simulink model "DDCU_wxt_v02_forA_LabviewV01"  (R2014a)
settings: Solver=FixedStepDiscrete  StartTime=0.0  StopTime=50  FixedStep=0.0005  RelTol=1e-3
InitFcn:
  | Veh_Par_wxt
values from neighbouring files (symbols this model uses):
  ag_thr = 0.4*g    (= 3.924)    [Veh_Par_wxt.m]
  B = 2.25    [Veh_Par_wxt.m]
  bra_pre_em = 12    [Veh_Par_wxt.m]
  bra_pre_gz2 = 12/3    (= 4)    [Veh_Par_wxt.m]
  bra_pre_gz34 = 12/3    (= 4)    [Veh_Par_wxt.m]
  bra_pre_yd = 12/2    (= 6)    [Veh_Par_wxt.m]
  brakepre_dem_data = [0 1 2 3 4 5 6 7 8 9 10 11 12]    [Veh_Par_wxt.m]
  brakeTrq_dem_data = [0 218.198 436.396 654.594 872.792 1090.99 1309.188 1527.386 1745.584 1963.782 2181.98 2400.178 2618.376]    [Veh_Par_wxt.m]
  bratrq_max = 4*2618.376    (= 10473.504)    [Veh_Par_wxt.m]
  eff_tran = 0.75    [Veh_Par_wxt.m]
  G = Mass*g    (= 36297)    [Veh_Par_wxt.m]
  kd1 = 1    [Veh_Par_wxt.m]
  kd2 = 1    [Veh_Par_wxt.m]
  kd3 = 1    [Veh_Par_wxt.m]
  ki1 = 1    [Veh_Par_wxt.m]
  ki2 = 1    [Veh_Par_wxt.m]
  ki3 = 1    [Veh_Par_wxt.m]
  kp1 = 1    [Veh_Par_wxt.m]
  kp2 = 1    [Veh_Par_wxt.m]
  kp3 = 1    [Veh_Par_wxt.m]
  L = 3.12    [Veh_Par_wxt.m]
  premax = 12    [Veh_Par_wxt.m]
  Radius = 0.20    (= 0.2)    [Veh_Par_wxt.m]
  s_opt_yi_add = 0.05    [Veh_Par_wxt.m]
  s_opt_zhuan_add = 0.05    [Veh_Par_wxt.m]
  spd_map_mot = [0 100 200 300 360 400 500 600 700 800 900]*tras_ratio    [Veh_Par_wxt.m]
  spdmax = 900*tras_ratio    (= 5580)    [Veh_Par_wxt.m]
  speed_thr_park = 5/3.6/Radius*30/pi    (= 66.3145596216)    [Veh_Par_wxt.m]
  tras_ratio = 6.2    [Veh_Par_wxt.m]
  trq_map_mot = [1200 1200 1200 1200 1200 1080 864 720 617 540 480]/tras_ratio    [Veh_Par_wxt.m]
  trqmax = 80    [Veh_Par_wxt.m]
  v_thr1_b = 5    [Veh_Par_wxt.m]
  v_thr2_b = 20    [Veh_Par_wxt.m]
  v_thr_park = 5    [Veh_Par_wxt.m]
undefined symbols (not defined in the file or in its folder): DiscIntNeverNeededParam
libraries: simulink x169, ec5744lib x9
(part 1 of 13)
settings Model: Creator=wxt  LastModifiedBy=wxt
settings OptimizationCC: InlineParams=on  InlineInvariantSignals=on  ExpressionFolding=off  RollThreshold=9  StateBitsets=on  DataBitsets=on  UseTempVars=on  ZeroExternalMemoryAtStartup=off  ZeroInternalMemoryAtStartup=off  EfficientFloat2IntCast=on  OptimizeModelRefInitCode=on  LifeSpan=1
settings DebuggingCC: InheritedTsInSrcMsg=none
settings HardwareCC: ProdLargestAtomicInteger=Long  ProdLargestAtomicFloat=Double  ProdIntDivRoundTo=Zero  ProdEndianess=BigEndian  ProdHWDeviceType=Freescale MPC5500
settings RTWCC: SystemTargetFile=ec5744.tlc  MakeCommand=make_rtw optimized_fixed_point=1  GenerateMakefile=off  TemplateMakefile=ec5744_lcc.tmf  PostCodeGenCommand=ec5744_pst_s2(buildInfo)  Description=Target for EC5744  GenerateReport=on  ProcessScript=ec5744_make_rtw_hook  IncludeHyperlinkInReport=on  LaunchReport=on
settings CodeAppCC: IgnoreCustomStorageClasses=off
settings STFCustomTargetCC: ModelReferenceCompliant=off  ConcurrentExecutionCompliant=off  IncludeMdlTerminateFcn=off  GeneratePreprocessorConditionals=Use local settings  CombineOutputUpdateFcns=on  SuppressErrorStatus=on  ERTCustomFileBanners=on  SupportContinuousTime=off  SupportNonInlinedSFcns=off  MATLABClassNameForMDSCustomization=Simulink.SoftwareTarget.ERTCustomization  GRTInterface=off  SystemTargetFile=ec5744.tlc
settings ERTTargetCC: GenerateSampleERTMain=off  ModelReferenceCompliant=off  IncludeMdlTerminateFcn=off  SuppressErrorStatus=on  GenerateASAP2=on  ERTSrcFileBannerTemplate=ec5744_code_template.cgt  ERTHdrFileBannerTemplate=ec5744_code_template.cgt  ERTDataSrcFileTemplate=ec5744_code_template.cgt  ERTDataHdrFileTemplate=ec5744_code_template.cgt  ERTCustomFileTemplate=ec5744_file_process.tlc

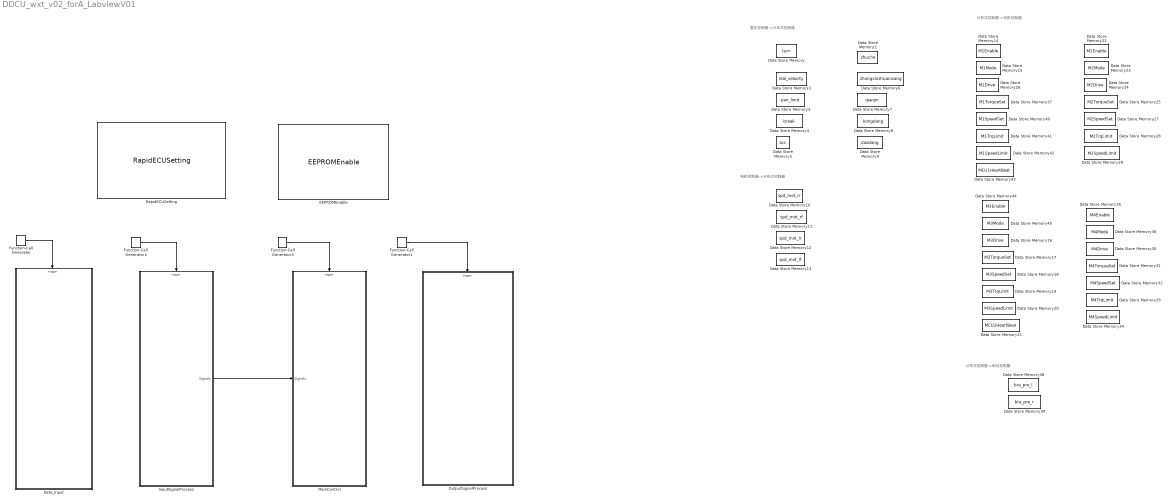
== system DDCU_wxt_v02_forA_LabviewV01 ==
  note: 电机控制器->分布式控制器
  note: 整车控制器->分布式控制器
  note: 分布式控制器->制动控制器
  note: 分布式控制器->电机控制器
  Data Store Memory : DataStoreMemory  DataStoreName=turn  ReadBeforeWriteMsg=warning  WriteAfterWriteMsg=warning  WriteAfterReadMsg=warning
  Data Store Memory1 : DataStoreMemory  DataStoreName=real_velocity  ReadBeforeWriteMsg=warning  WriteAfterWriteMsg=warning  WriteAfterReadMsg=warning
  Data Store Memory10 : DataStoreMemory  DataStoreName=spd_mot_rr  ReadBeforeWriteMsg=warning  WriteAfterWriteMsg=warning  WriteAfterReadMsg=warning
  Data Store Memory11 : DataStoreMemory  DataStoreName=spd_mot_rf  ReadBeforeWriteMsg=warning  WriteAfterWriteMsg=warning  WriteAfterReadMsg=warning
  Data Store Memory12 : DataStoreMemory  DataStoreName=spd_mot_lr  ReadBeforeWriteMsg=warning  WriteAfterWriteMsg=warning  WriteAfterReadMsg=warning
  Data Store Memory13 : DataStoreMemory  DataStoreName=spd_mot_lf  ReadBeforeWriteMsg=warning  WriteAfterWriteMsg=warning  WriteAfterReadMsg=warning
  Data Store Memory14 : DataStoreMemory  DataStoreName=M1Enable  ReadBeforeWriteMsg=warning  WriteAfterWriteMsg=warning  WriteAfterReadMsg=warning
  Data Store Memory15 : DataStoreMemory  DataStoreName=M1Mode  ReadBeforeWriteMsg=warning  WriteAfterWriteMsg=warning  WriteAfterReadMsg=warning
  Data Store Memory16 : DataStoreMemory  DataStoreName=M3Drive  ReadBeforeWriteMsg=warning  WriteAfterWriteMsg=warning  WriteAfterReadMsg=warning
  Data Store Memory17 : DataStoreMemory  DataStoreName=M3TorqueSet  ReadBeforeWriteMsg=warning  WriteAfterWriteMsg=warning  WriteAfterReadMsg=warning
  Data Store Memory18 : DataStoreMemory  DataStoreName=M3SpeedSet  ReadBeforeWriteMsg=warning  WriteAfterWriteMsg=warning  WriteAfterReadMsg=warning
  Data Store Memory19 : DataStoreMemory  DataStoreName=M3TrqLimit  ReadBeforeWriteMsg=warning  WriteAfterWriteMsg=warning  WriteAfterReadMsg=warning
  Data Store Memory2 : DataStoreMemory  DataStoreName=zhuche  ReadBeforeWriteMsg=warning  WriteAfterWriteMsg=warning  WriteAfterReadMsg=warning
  Data Store Memory20 : DataStoreMemory  DataStoreName=M3SpeedLimit  ReadBeforeWriteMsg=warning  WriteAfterWriteMsg=warning  WriteAfterReadMsg=warning
  Data Store Memory21 : DataStoreMemory  DataStoreName=MCU2HeartBeat  ReadBeforeWriteMsg=warning  WriteAfterWriteMsg=warning  WriteAfterReadMsg=warning
  Data Store Memory22 : DataStoreMemory  DataStoreName=M2Enable  ReadBeforeWriteMsg=warning  WriteAfterWriteMsg=warning  WriteAfterReadMsg=warning
  Data Store Memory23 : DataStoreMemory  DataStoreName=M2Mode  ReadBeforeWriteMsg=warning  WriteAfterWriteMsg=warning  WriteAfterReadMsg=warning
  Data Store Memory24 : DataStoreMemory  DataStoreName=M2Drive  ReadBeforeWriteMsg=warning  WriteAfterWriteMsg=warning  WriteAfterReadMsg=warning
  Data Store Memory25 : DataStoreMemory  DataStoreName=M2TorqueSet  ReadBeforeWriteMsg=warning  WriteAfterWriteMsg=warning  WriteAfterReadMsg=warning
  Data Store Memory26 : DataStoreMemory  DataStoreName=M1Drive  ReadBeforeWriteMsg=warning  WriteAfterWriteMsg=warning  WriteAfterReadMsg=warning
  Data Store Memory27 : DataStoreMemory  DataStoreName=M2SpeedSet  ReadBeforeWriteMsg=warning  WriteAfterWriteMsg=warning  WriteAfterReadMsg=warning
  Data Store Memory28 : DataStoreMemory  DataStoreName=M2TrqLimit  ReadBeforeWriteMsg=warning  WriteAfterWriteMsg=warning  WriteAfterReadMsg=warning
  Data Store Memory29 : DataStoreMemory  DataStoreName=M2SpeedLimit  ReadBeforeWriteMsg=warning  WriteAfterWriteMsg=warning  WriteAfterReadMsg=warning
  Data Store Memory3 : DataStoreMemory  DataStoreName=pwr_limit  ReadBeforeWriteMsg=warning  WriteAfterWriteMsg=warning  WriteAfterReadMsg=warning
  Data Store Memory30 : DataStoreMemory  DataStoreName=M4Drive  ReadBeforeWriteMsg=warning  WriteAfterWriteMsg=warning  WriteAfterReadMsg=warning
  Data Store Memory31 : DataStoreMemory  DataStoreName=M4TorqueSet  ReadBeforeWriteMsg=warning  WriteAfterWriteMsg=warning  WriteAfterReadMsg=warning
  Data Store Memory32 : DataStoreMemory  DataStoreName=M4SpeedSet  ReadBeforeWriteMsg=warning  WriteAfterWriteMsg=warning  WriteAfterReadMsg=warning
  Data Store Memory33 : DataStoreMemory  DataStoreName=M4TrqLimit  ReadBeforeWriteMsg=warning  WriteAfterWriteMsg=warning  WriteAfterReadMsg=warning
  Data Store Memory34 : DataStoreMemory  DataStoreName=M4SpeedLimit  ReadBeforeWriteMsg=warning  WriteAfterWriteMsg=warning  WriteAfterReadMsg=warning
  Data Store Memory35 : DataStoreMemory  DataStoreName=M4Enable  ReadBeforeWriteMsg=warning  WriteAfterWriteMsg=warning  WriteAfterReadMsg=warning
  Data Store Memory36 : DataStoreMemory  DataStoreName=M4Mode  ReadBeforeWriteMsg=warning  WriteAfterWriteMsg=warning  WriteAfterReadMsg=warning
  Data Store Memory37 : DataStoreMemory  DataStoreName=M1TorqueSet  ReadBeforeWriteMsg=warning  WriteAfterWriteMsg=warning  WriteAfterReadMsg=warning
  Data Store Memory38 : DataStoreMemory  DataStoreName=bra_pre_l  ReadBeforeWriteMsg=warning  WriteAfterWriteMsg=warning  WriteAfterReadMsg=warning
  Data Store Memory39 : DataStoreMemory  DataStoreName=bra_pre_r  ReadBeforeWriteMsg=warning  WriteAfterWriteMsg=warning  WriteAfterReadMsg=warning
  Data Store Memory4 : DataStoreMemory  DataStoreName=break  ReadBeforeWriteMsg=warning  WriteAfterWriteMsg=warning  WriteAfterReadMsg=warning
  Data Store Memory40 : DataStoreMemory  DataStoreName=M1SpeedSet  ReadBeforeWriteMsg=warning  WriteAfterWriteMsg=warning  WriteAfterReadMsg=warning
  Data Store Memory41 : DataStoreMemory  DataStoreName=M1TrqLimit  ReadBeforeWriteMsg=warning  WriteAfterWriteMsg=warning  WriteAfterReadMsg=warning
  Data Store Memory42 : DataStoreMemory  DataStoreName=M1SpeedLimit  ReadBeforeWriteMsg=warning  WriteAfterWriteMsg=warning  WriteAfterReadMsg=warning
  Data Store Memory43 : DataStoreMemory  DataStoreName=MCU1HeartBeat  ReadBeforeWriteMsg=warning  WriteAfterWriteMsg=warning  WriteAfterReadMsg=warning
  Data Store Memory44 : DataStoreMemory  DataStoreName=M3Enable  ReadBeforeWriteMsg=warning  WriteAfterWriteMsg=warning  WriteAfterReadMsg=warning
  Data Store Memory45 : DataStoreMemory  DataStoreName=M3Mode  ReadBeforeWriteMsg=warning  WriteAfterWriteMsg=warning  WriteAfterReadMsg=warning
  Data Store Memory5 : DataStoreMemory  DataStoreName=acc  ReadBeforeWriteMsg=warning  WriteAfterWriteMsg=warning  WriteAfterReadMsg=warning
  Data Store Memory6 : DataStoreMemory  DataStoreName=zhongxinzhuanxiang  ReadBeforeWriteMsg=warning  WriteAfterWriteMsg=warning  WriteAfterReadMsg=warning
  Data Store Memory7 : DataStoreMemory  DataStoreName=qianjin  ReadBeforeWriteMsg=warning  WriteAfterWriteMsg=warning  WriteAfterReadMsg=warning
  Data Store Memory8 : DataStoreMemory  DataStoreName=kongdang  ReadBeforeWriteMsg=warning  WriteAfterWriteMsg=warning  WriteAfterReadMsg=warning
  Data Store Memory9 : DataStoreMemory  DataStoreName=daodang  ReadBeforeWriteMsg=warning  WriteAfterWriteMsg=warning  WriteAfterReadMsg=warning
  Data_Input : Subsystem  TreatAsAtomicUnit=on
  EEPROMEnable : ec5744lib/RapidECU_U3/09MemoryManagement/EEPROMEnable  eepromenable=on
  Function-Call Generator{,1..3} (4 alike) : simulink/Ports & Subsystems/Function-Call Generator  sample_time=0.05  numberOfIterations=1
  InputSignalProcess : Subsystem
  MainControl : Subsystem
  OutputSignalProcess : Subsystem  TreatAsAtomicUnit=on
  RapidECUSetting : ec5744lib/RapidECU_U3/RapidECUSetting
      link override CAN: apdf=4  bpdf=4  cpdf=4  acmt=Extended(29-bit ID)  bcmt=Extended(29-bit ID)
      link override LIN: abrt=19200
  wires:
  Function-Call Generator/1 -> Data_Input/Trigger
  Function-Call Generator1/1 -> OutputSignalProcess/Trigger
  Function-Call Generator2/1 -> InputSignalProcess/Trigger
  InputSignalProcess/1(Signals) -> MainControl/1(Signals)
  Function-Call Generator3/1 -> MainControl/Trigger

== system DDCU_wxt_v02_forA_LabviewV01/Data_Input ==
  note: 电机控制器->分布式控制器
  note: 整车控制器->分布式控制器
  function : TriggerPort  TriggerType=function-call
  CANReceive : ec5744lib/RapidECU_U3/04CANCommunication/CANReceive  canmodule=0  canbuffer=0  canmessageid=hex2dec('1502C23A')  canmessagetype=Extended(29-bit ID)  datalength=8  sampletime=-1
  CANReceive1 : ec5744lib/RapidECU_U3/04CANCommunication/CANReceive  canmodule=0  canbuffer=1  canmessageid=hex2dec('0902C23A')  canmessagetype=Extended(29-bit ID)  datalength=8  sampletime=-1
  CANReceive2 : ec5744lib/RapidECU_U3/04CANCommunication/CANReceive  canmodule=0  canbuffer=2  canmessageid=hex2dec('0C0101F0')  canmessagetype=Extended(29-bit ID)  datalength=8  sampletime=-1
  Data Store Write : DataStoreWrite  DataStoreName=turn  DataStoreElements=turn
  Data Store Write1 : DataStoreWrite  DataStoreName=real_velocity
  Data Store Write10 : DataStoreWrite  DataStoreName=spd_mot_rr
  Data Store Write11 : DataStoreWrite  DataStoreName=spd_mot_rf
  Data Store Write12 : DataStoreWrite  DataStoreName=spd_mot_lr
  Data Store Write13 : DataStoreWrite  DialogController=Simulink.DDGSource  DataStoreName=spd_mot_lf  DataStoreElements=spd_mot_lf
  Data Store Write2 : DataStoreWrite  DataStoreName=pwr_limit
  Data Store Write3 : DataStoreWrite  DataStoreName=break
  Data Store Write4 : DataStoreWrite  DataStoreName=acc
  Data Store Write5 : DataStoreWrite  DataStoreName=zhuche
  Data Store Write6 : DataStoreWrite  DataStoreName=zhongxinzhuanxiang
  Data Store Write7 : DataStoreWrite  DataStoreName=qianjin
  Data Store Write8 : DataStoreWrite  DataStoreName=kongdang
  Data Store Write9 : DataStoreWrite  DataStoreName=daodang
  HCU1_VCU : Subsystem  TreatAsAtomicUnit=on
  HCU1_VCU1 : Subsystem  TreatAsAtomicUnit=on
  HCU2_VCU : Subsystem  TreatAsAtomicUnit=on
  Terminator{,1..5} (6 alike) : Terminator
  wires:
  CANReceive/1 -> HCU1_VCU/Trigger
  CANReceive/2 -> HCU1_VCU/1(In1)
  CANReceive/4 -> HCU1_VCU/2(In2)
  CANReceive/3 -> Terminator/1
  CANReceive/5 -> Terminator1/1
  HCU1_VCU/3(pwr_limit) -> Data Store Write2/1
  HCU1_VCU/2(real_velocity) -> Data Store Write1/1
  HCU1_VCU/4(break) -> Data Store Write3/1
  HCU1_VCU/1(turn) -> Data Store Write/1
  HCU1_VCU/5(acc) -> Data Store Write4/1
  CANReceive1/1 -> HCU2_VCU/Trigger
  CANReceive1/2 -> HCU2_VCU/1(In1)
  CANReceive1/4 -> HCU2_VCU/2(In2)
  CANReceive1/3 -> Terminator2/1
  CANReceive1/5 -> Terminator3/1
  HCU2_VCU/3(qianjin) -> Data Store Write7/1
  HCU2_VCU/4(kongdang) -> Data Store Write8/1
  HCU2_VCU/2(zhongxinzhuanxiang) -> Data Store Write6/1
  HCU2_VCU/1(zhuche) -> Data Store Write5/1
  HCU2_VCU/5(daodang) -> Data Store Write9/1
  CANReceive2/1 -> HCU1_VCU1/Trigger
  CANReceive2/2 -> HCU1_VCU1/1(In1)
  CANReceive2/4 -> HCU1_VCU1/2(In2)
  CANReceive2/3 -> Terminator4/1
  CANReceive2/5 -> Terminator5/1
  HCU1_VCU1/1(spd_mot_rr) -> Data Store Write10/1
  HCU1_VCU1/2(spd_mot_rf) -> Data Store Write11/1
  HCU1_VCU1/3(spd_mot_lr) -> Data Store Write12/1
  HCU1_VCU1/4(spd_mot_lf) -> Data Store Write13/1

== system DDCU_wxt_v02_forA_LabviewV01/InputSignalProcess ==
  note: 注：所有的单位转换都发生在此模块
      | 速度 km/h
      | 角速度 rpm
      | 加速度信号0-100
      | 制动信号0-100
      | 向左为正
      | 同时包括信号的一些简单处理，如根究摇杆位置，判断所需档位等
  function : TriggerPort  TriggerType=function-call
  Battery : Subsystem
  BraSystem : Subsystem
  Bus Creator : BusCreator  Inputs=6
  Constant{,1..3,6..8,15,17} (9 alike) : Constant  Value=0
  Constant{4..5,10,12} (4 alike) : Constant  Value=1000
  Constant{11,13..14,16} (4 alike) : Constant  Value=-1000
  Constant9 : Constant  Value=-80
  Data Store Read : DataStoreRead  DialogController=Simulink.DDGSource  DataStoreName=turn  DataStoreElements=turn
  Data Store Read1 : DataStoreRead  DataStoreName=pwr_limit
  Data Store Read10 : DataStoreRead  DataStoreName=spd_mot_rr
  Data Store Read11 : DataStoreRead  DataStoreName=spd_mot_rf
  Data Store Read12 : DataStoreRead  DataStoreName=spd_mot_lr
  Data Store Read13 : DataStoreRead  DataStoreName=spd_mot_lf  DataStoreElements=spd_mot_lf
  Data Store Read2 : DataStoreRead  DataStoreName=break
  Data Store Read3 : DataStoreRead  DataStoreName=acc
  Data Store Read4 : DataStoreRead  DataStoreName=real_velocity
  Data Store Read5 : DataStoreRead  DataStoreName=zhuche
  Data Store Read6 : DataStoreRead  DataStoreName=zhongxinzhuanxiang
  Data Store Read7 : DataStoreRead  DataStoreName=qianjin
  Data Store Read8 : DataStoreRead  DataStoreName=kongdang
  Data Store Read9 : DataStoreRead  DataStoreName=daodang
  DriveMotor : Subsystem
  IMU : Subsystem
  Signal Conversion : SignalConversion
  Subsystem : Subsystem
  Suspension : Subsystem
  YaoKong : Subsystem
  Signals : Outport
  wires:
  DriveMotor/1(DriveMotor) -> Bus Creator/2
  BraSystem/1(BraPre) -> Bus Creator/3
  YaoKong/1(YaoKong_dem) -> Bus Creator/1
  IMU/1(IMU) -> Bus Creator/4
  Suspension/1(Center_of_Mass) -> Bus Creator/5
  Battery/1(Bat) -> Bus Creator/6
  Constant8/1 -> Suspension/1(location_center)
  Constant9/1 -> Battery/2(pwr_chg_bat)
  Data Store Read1/1 -> Battery/1(pwr_dis_bat)  "pwr_limit"
  Data Store Read6/1 -> Subsystem/2(zhongxinzhuanxiang)  "zhongxinzhuanxiang"
  Data Store Read7/1 -> Subsystem/3(qianjin)  "qianjin"
  Data Store Read8/1 -> Subsystem/4(kongdang)  "kongdang"
  Data Store Read9/1 -> Subsystem/5(daodang)  "daodang"
  Subsystem/1(mode_dem) -> YaoKong/1(mode_dem)  "mode_dem"
  Data Store Read3/1 -> YaoKong/2(acc_dem)  "acc"
  Data Store Read/1 -> YaoKong/3(steer_dem)  "turn"
  Data Store Read2/1 -> YaoKong/4(brake_dem)  "breakyg"
  Data Store Read4/1 -> IMU/1(v_act)  "real_velocity"
  Data Store Read10/1 -> DriveMotor/16(speed_act_rr)  "spd_mot_rr"
  Data Store Read11/1 -> DriveMotor/11(speed_act_rf)  "spd_mot_rf"
  Data Store Read12/1 -> DriveMotor/6(speed_act_lr)  "spd_mot_lr"
  Data Store Read13/1 -> DriveMotor/1(speed_act_lf)  "spd_mot_lf"
  Bus Creator/1 -> Signal Conversion/1
  Constant/1 -> YaoKong/5(brake_emerg)
  Constant1/1 -> YaoKong/6(HAC)
  Constant6/1 -> BraSystem/2(BraPre_act_r), BraSystem/1(BraPre_act_l)
  Constant7/1 -> IMU/3(dis_north), IMU/4(dis_sky), IMU/5(hangxiangangle), IMU/6(fuyangangle), IMU/7(henggunangle), IMU/8(acc_x), IMU/9(acc_y), IMU/10(acc_z), IMU/11(jiaosudu_x), IMU/12(jiaosudu_y), IMU/13(jiaosudu_z), IMU/2(dis_east)
  Data Store Read5/1 -> Subsystem/1(zhuche)  "zhuche"
  Signal Conversion/1 -> Signals/1
  Constant2/1 -> DriveMotor/5(guzhang_lf)
  Constant10/1 -> DriveMotor/3(trqlimU_dig_lf)
  Constant11/1 -> DriveMotor/4(trqlimL_dig_lf)
  Constant3/1 -> DriveMotor/10(guzhang_lr)
  Constant12/1 -> DriveMotor/8(trqlimU_dig_lr)
  Constant13/1 -> DriveMotor/9(trqlimL_dig_lr)
  Constant15/1 -> DriveMotor/15(guzhang_rf)
  Constant4/1 -> DriveMotor/13(trqlimU_dig_rf)
  Constant14/1 -> DriveMotor/14(trqlimL_dig_rf)
  Constant17/1 -> DriveMotor/20(guzhang_rr)
  Constant5/1 -> DriveMotor/18(trqlimU_dig_rr)
  Constant16/1 -> DriveMotor/19(trqlimL_dig_rr)

== system DDCU_wxt_v02_forA_LabviewV01/MainControl ==
  Signals : Inport
  function : TriggerPort  TriggerType=function-call
  Scope : Scope
      settings: TimeRange=20  YMin=4  SaveName=ScopeData53
  SendOutPrepare : Subsystem
  To Workspace : ToWorkspace  VariableName=simout5  SaveFormat=Timeseries  SampleTime=-1
  mode_control : Subsystem
  mode_switch : Subsystem
  wires:
  Signals/1 -> mode_control/2(Signals), mode_switch/1(Signals)
  mode_switch/1(mode_dem_out) -> mode_control/1(mode_dem_out), Scope/1, To Workspace/1
  mode_control/1(com_dem) -> SendOutPrepare/1(com_dem)

== system DDCU_wxt_v02_forA_LabviewV01/OutputSignalProcess ==
  function : TriggerPort  TriggerType=function-call
  CANTransmit : ec5744lib/RapidECU_U3/04CANCommunication/CANTransmit  canmodule=0  canbuffer=8  canmessageid=hex2dec('0C01F001')  canmessagetype=Extended(29-bit ID)  datalength=8  sampletime=-1
  CANTransmit1 : ec5744lib/RapidECU_U3/04CANCommunication/CANTransmit  canmodule=0  canbuffer=9  canmessageid=hex2dec('0C01F002')  canmessagetype=Extended(29-bit ID)  datalength=8  sampletime=-1
  CANTransmit2 : ec5744lib/RapidECU_U3/04CANCommunication/CANTransmit  canmodule=0  canbuffer=10  canmessageid=hex2dec('804623A')  canmessagetype=Extended(29-bit ID)  datalength=8  sampletime=-1
  CANTransmit3 : ec5744lib/RapidECU_U3/04CANCommunication/CANTransmit  canmodule=0  canbuffer=11  canmessageid=hex2dec('0CF6EAF0')  canmessagetype=Extended(29-bit ID)  datalength=8  sampletime=-1
  Data Store Read : DataStoreRead  DataStoreName=M1Enable
  Data Store Read1 : DataStoreRead  DataStoreName=M1Mode
  Data Store Read10 : DataStoreRead  DataStoreName=M3Drive
  Data Store Read11 : DataStoreRead  DataStoreName=M3TorqueSet
  Data Store Read12 : DataStoreRead  DataStoreName=M3SpeedSet
  Data Store Read13 : DataStoreRead  DialogController=Simulink.DDGSource  DataStoreName=M3TrqLimit
  Data Store Read14 : DataStoreRead  DataStoreName=M3SpeedLimit
  Data Store Read15 : DataStoreRead  DataStoreName=MCU2HeartBeat
  Data Store Read16 : DataStoreRead  DataStoreName=M2Enable
  Data Store Read17 : DataStoreRead  DataStoreName=M2Mode
  Data Store Read18 : DataStoreRead  DataStoreName=M2Drive
  Data Store Read19 : DataStoreRead  DataStoreName=M2TorqueSet
  Data Store Read2 : DataStoreRead  DataStoreName=M1Drive
  Data Store Read20 : DataStoreRead  DataStoreName=M2SpeedSet
  Data Store Read21 : DataStoreRead  DataStoreName=M2TrqLimit
  Data Store Read22 : DataStoreRead  DataStoreName=M2SpeedLimit
  Data Store Read23 : DataStoreRead  DataStoreName=M4Drive
  Data Store Read24 : DataStoreRead  DataStoreName=M4TorqueSet
  Data Store Read25 : DataStoreRead  DataStoreName=M4SpeedSet
  Data Store Read26 : DataStoreRead  DataStoreName=M4TrqLimit
  Data Store Read27 : DataStoreRead  DataStoreName=M4SpeedLimit
  Data Store Read28 : DataStoreRead  DataStoreName=M4Enable
  Data Store Read29 : DataStoreRead  DataStoreName=M4Mode
  Data Store Read3 : DataStoreRead  DataStoreName=M1TorqueSet
  Data Store Read30 : DataStoreRead  DataStoreName=bra_pre_l
  Data Store Read31 : DataStoreRead  DataStoreName=bra_pre_r
  Data Store Read4 : DataStoreRead  DataStoreName=M1SpeedSet
  Data Store Read5 : DataStoreRead  DataStoreName=M1TrqLimit
  Data Store Read6 : DataStoreRead  DataStoreName=M1SpeedLimit
  Data Store Read7 : DataStoreRead  DataStoreName=MCU1HeartBeat
  Data Store Read8 : DataStoreRead  DataStoreName=M3Enable
  Data Store Read9 : DataStoreRead  DataStoreName=M3Mode
  Ground : Ground
  Ground1 : Ground
  Ground2 : Ground
  Terminator{,1..11} (12 alike) : Terminator
  VCU_ESC : Subsystem
  VCU_MCU1 : Subsystem
  VCU_MCU1_replace : Subsystem  Commented=on
  VCU_MCU2 : Subsystem
  VCU_MCU2_replace : Subsystem  Commented=on
  VCU_Park : Subsystem
  wires:
  Ground/1 -> VCU_Park/1(ParkEnable_in)
  Ground1/1 -> VCU_ESC/1(VVMS_BrkSts_flg_in)
  Ground2/1 -> VCU_ESC/2(VVMS_ParkSts_flg_in)
  VCU_MCU1/1(output) -> CANTransmit/1
  CANTransmit/1 -> Terminator/1
  VCU_MCU2/1(output) -> CANTransmit1/1
  CANTransmit1/1 -> Terminator1/1
  VCU_Park/1(output) -> CANTransmit2/1
  CANTransmit2/1 -> Terminator2/1
  VCU_ESC/1(output) -> CANTransmit3/1
  CANTransmit3/1 -> Terminator3/1
  Data Store Read4/1 -> Terminator4/1
  Data Store Read5/1 -> Terminator5/1
  Data Store Read20/1 -> Terminator6/1
  Data Store Read21/1 -> Terminator7/1
  Data Store Read12/1 -> Terminator8/1
  Data Store Read13/1 -> Terminator9/1
  Data Store Read25/1 -> Terminator10/1
  Data Store Read26/1 -> Terminator11/1
  Data Store Read7/1 -> VCU_MCU1/11(MCU1HeartBeat_in)
  Data Store Read19/1 -> VCU_MCU1/9(M2TorqueSet_in)  "M2TorqueSet"
  Data Store Read22/1 -> VCU_MCU1/10(M2SpeedLimit_in)
  Data Store Read6/1 -> VCU_MCU1/5(M1SpeedLimit_in)
  Data Store Read3/1 -> VCU_MCU1/4(M1TorqueSet_in)  "M1TorqueSet"
  Data Store Read16/1 -> VCU_MCU1/6(M2Enable_in)
  Data Store Read17/1 -> VCU_MCU1/7(M2Mode_in)
  Data Store Read18/1 -> VCU_MCU1/8(M2Drive_in)
  Data Store Read/1 -> VCU_MCU1/1(M1Enable_in)
  Data Store Read2/1 -> VCU_MCU1/3(M1Drive_in)
  Data Store Read1/1 -> VCU_MCU1/2(M1Mode_in)
  Data Store Read14/1 -> VCU_MCU2/5(M3SpeedLimit_in)
  Data Store Read11/1 -> VCU_MCU2/4(M3TorqueSet_in)  "M3TorqueSet"
  Data Store Read15/1 -> VCU_MCU2/11(MCU2HeartBeat_in)
  Data Store Read27/1 -> VCU_MCU2/10(M4SpeedLimit_in)
  Data Store Read10/1 -> VCU_MCU2/3(M3Drive_in)
  Data Store Read8/1 -> VCU_MCU2/1(M3Enable_in)
  Data Store Read9/1 -> VCU_MCU2/2(M3Mode_in)
  Data Store Read28/1 -> VCU_MCU2/6(M4Enable_in)
  Data Store Read24/1 -> VCU_MCU2/9(M4TorqueSet_in)  "M4TorqueSet"
  Data Store Read23/1 -> VCU_MCU2/8(M4Drive_in)
  Data Store Read29/1 -> VCU_MCU2/7(M4Mode_in)
  Data Store Read31/1 -> VCU_ESC/4(VVMS_BrkPSetRi_MPa_in)  "bra_pre_r"
  Data Store Read30/1 -> VCU_ESC/3(VVMS_BrkPSetLe_MPa_in)  "bra_pre_l"

== system DDCU_wxt_v02_forA_LabviewV01/Data_Input/HCU1_VCU ==
  In1 : Inport
  In2 : Inport  Port=2
  function : TriggerPort  TriggerType=function-call
  HCU1_VCU : Subsystem
  turn : Outport
  real_velocity : Outport  Port=2
  pwr_limit : Outport  Port=3
  break : Outport  Port=4
  acc : Outport  Port=5
  wires:
  In1/1 -> HCU1_VCU/Enable
  In2/1 -> HCU1_VCU/1(input)
  HCU1_VCU/3(pwr_limit_Out) -> pwr_limit/1
  HCU1_VCU/4(break_Out) -> break/1
  HCU1_VCU/2(real_velocity_Out) -> real_velocity/1
  HCU1_VCU/5(acc_Out) -> acc/1
  HCU1_VCU/1(turn_Out) -> turn/1

== system DDCU_wxt_v02_forA_LabviewV01/Data_Input/HCU1_VCU1 ==
  In1 : Inport
  In2 : Inport  Port=2
  function : TriggerPort  TriggerType=function-call
  MUC1_VCU1 : Subsystem
  spd_mot_rr : Outport
  spd_mot_rf : Outport  Port=2
  spd_mot_lr : Outport  Port=3
  spd_mot_lf : Outport  Port=4
  wires:
  In2/1 -> MUC1_VCU1/1(input)
  In1/1 -> MUC1_VCU1/Enable
  MUC1_VCU1/2(spd_mot_rf_Out) -> spd_mot_rf/1
  MUC1_VCU1/1(spd_mot_rr_Out) -> spd_mot_rr/1
  MUC1_VCU1/3(spd_mot_lr_Out) -> spd_mot_lr/1
  MUC1_VCU1/4(spd_mot_lf_Out) -> spd_mot_lf/1

== system DDCU_wxt_v02_forA_LabviewV01/Data_Input/HCU2_VCU ==
  In1 : Inport
  In2 : Inport  Port=2
  function : TriggerPort  TriggerType=function-call
  HCU2_VCU : Subsystem
  zhuche : Outport
  zhongxinzhuanxiang : Outport  Port=2
  qianjin : Outport  Port=3
  kongdang : Outport  Port=4
  daodang : Outport  Port=5
  wires:
  In2/1 -> HCU2_VCU/1(input)
  In1/1 -> HCU2_VCU/Enable
  HCU2_VCU/2(zhongxinzhuanxiang_Out) -> zhongxinzhuanxiang/1
  HCU2_VCU/3(qianjin_Out) -> qianjin/1
  HCU2_VCU/1(zhuche_Out) -> zhuche/1
  HCU2_VCU/4(kongdang_Out) -> kongdang/1
  HCU2_VCU/5(daodang_Out) -> daodang/1

== system DDCU_wxt_v02_forA_LabviewV01/InputSignalProcess/Battery ==
  pwr_dis_bat : Inport
  pwr_chg_bat : Inport  Port=2
  Bus Creator : BusCreator  Inputs=2
  Bat : Outport
  wires:
  pwr_dis_bat/1 -> Bus Creator/1  "pwr_dis_bat"
  Bus Creator/1 -> Bat/1  "Bat"
  pwr_chg_bat/1 -> Bus Creator/2  "pwr_chg_bat"

== system DDCU_wxt_v02_forA_LabviewV01/InputSignalProcess/BraSystem ==
  BraPre_act_l : Inport
  BraPre_act_r : Inport  Port=2
  Bus Creator : BusCreator  Inputs=2
  BraPre : Outport
  wires:
  BraPre_act_l/1 -> Bus Creator/1  "BraPre_act"
  Bus Creator/1 -> BraPre/1  "BraPre"
  BraPre_act_r/1 -> Bus Creator/2  "BraPre_act_r"

== system DDCU_wxt_v02_forA_LabviewV01/InputSignalProcess/DriveMotor ==
  speed_act_lf : Inport
  trq_act_lf : Inport  Port=2
  trqlimU_dig_lf : Inport  Port=3
  trqlimL_dig_lf : Inport  Port=4
  guzhang_lf : Inport  Port=5
  speed_act_lr : Inport  Port=6
  trq_act_lr : Inport  Port=7
  trqlimU_dig_lr : Inport  Port=8
  trqlimL_dig_lr : Inport  Port=9
  guzhang_lr : Inport  Port=10
  speed_act_rf : Inport  Port=11
  trq_act_rf : Inport  Port=12
  trqlimU_dig_rf : Inport  Port=13
  trqlimL_dig_rf : Inport  Port=14
  guzhang_rf : Inport  Port=15
  speed_act_rr : Inport  Port=16
  trq_act_rr : Inport  Port=17
  trqlimU_dig_rr : Inport  Port=18
  trqlimL_dig_rr : Inport  Port=19
  guzhang_rr : Inport  Port=20
  Bus Creator : BusCreator  Inputs=20
  DriveMotor : Outport
  wires:
  Bus Creator/1 -> DriveMotor/1  "DriveMotor"
  trqlimL_dig_lr/1 -> Bus Creator/9  "trqlimL_dig_lr"
  trq_act_lf/1 -> Bus Creator/2  "trq_act_lf"
  trq_act_lr/1 -> Bus Creator/7  "trq_act_lr"
  trqlimL_dig_lf/1 -> Bus Creator/4  "trqlimL_dig_lf"
  trqlimU_dig_lf/1 -> Bus Creator/3  "trqlimU_dig_lf"
  trqlimU_dig_lr/1 -> Bus Creator/8  "trqlimU_dig_lr"
  speed_act_lf/1 -> Bus Creator/1  "speed_act_lf"
  speed_act_lr/1 -> Bus Creator/6  "speed_act_lr"
  guzhang_rf/1 -> Bus Creator/15  "guzhang_rf"
  guzhang_lf/1 -> Bus Creator/5  "guzhang_lf"
  guzhang_lr/1 -> Bus Creator/10  "guzhang_lr"
  speed_act_rf/1 -> Bus Creator/11  "speed_act_rf"
  guzhang_rr/1 -> Bus Creator/20  "guzhang_rr"
  trq_act_rf/1 -> Bus Creator/12  "trq_act_rf"
  speed_act_rr/1 -> Bus Creator/16  "speed_act_rr"
  trqlimL_dig_rf/1 -> Bus Creator/14  "trqlimL_dig_rf"
  trq_act_rr/1 -> Bus Creator/17  "trq_act_rr"
  trqlimL_dig_rr/1 -> Bus Creator/19  "trqlimL_dig_rr"
  trqlimU_dig_rf/1 -> Bus Creator/13  "trqlimU_dig_rf"
  trqlimU_dig_rr/1 -> Bus Creator/18  "trqlimU_dig_rr"

== system DDCU_wxt_v02_forA_LabviewV01/InputSignalProcess/IMU ==
  v_act : Inport
  dis_east : Inport  Port=2
  dis_north : Inport  Port=3
  dis_sky : Inport  Port=4
  hangxiangangle : Inport  Port=5
  fuyangangle : Inport  Port=6
  henggunangle : Inport  Port=7
  acc_x : Inport  Port=8
  acc_y : Inport  Port=9
  acc_z : Inport  Port=10
  jiaosudu_x : Inport  Port=11
  jiaosudu_y : Inport  Port=12
  jiaosudu_z : Inport  Port=13
  Bus Creator : BusCreator  Inputs=13
  IMU : Outport
  wires:
  Bus Creator/1 -> IMU/1  "IMU"
  dis_east/1 -> Bus Creator/2  "dis_east"
  hangxiangangle/1 -> Bus Creator/5  "hangxiangangle"
  dis_north/1 -> Bus Creator/3  "dis_north"
  dis_sky/1 -> Bus Creator/4  "dis_sky"
  fuyangangle/1 -> Bus Creator/6  "fuyangangle"
  acc_y/1 -> Bus Creator/9  "acc_y"
  henggunangle/1 -> Bus Creator/7  "henggunangle"
  acc_x/1 -> Bus Creator/8  "acc_x"
  acc_z/1 -> Bus Creator/10  "acc_z"
  jiaosudu_z/1 -> Bus Creator/13  "jiaosudu_z"
  jiaosudu_x/1 -> Bus Creator/11  "jiaosudu_x"
  jiaosudu_y/1 -> Bus Creator/12  "jiaosudu_y"
  v_act/1 -> Bus Creator/1  "v_act"

== system DDCU_wxt_v02_forA_LabviewV01/InputSignalProcess/Subsystem ==
  zhuche : Inport
  zhongxinzhuanxiang : Inport  Port=2
  qianjin : Inport  Port=3
  kongdang : Inport  Port=4
  daodang : Inport  Port=5
  MATLAB Function : MATLAB Function  TreatAsAtomicUnit=on
  mode_dem : Outport
  wires:
  MATLAB Function/1(mode_dem) -> mode_dem/1
  zhuche/1 -> MATLAB Function/1(zhuche)
  zhongxinzhuanxiang/1 -> MATLAB Function/2(zhongxinzhuanxiang)
  qianjin/1 -> MATLAB Function/3(qianjin)
  kongdang/1 -> MATLAB Function/4(kongdang)
  daodang/1 -> MATLAB Function/5(daodang)

== system DDCU_wxt_v02_forA_LabviewV01/InputSignalProcess/Suspension ==
  location_center : Inport
  Bus Creator : BusCreator  Inputs=1
  Center_of_Mass : Outport
  wires:
  Bus Creator/1 -> Center_of_Mass/1  "Center_of_Mass"
  location_center/1 -> Bus Creator/1  "location_center"

== system DDCU_wxt_v02_forA_LabviewV01/InputSignalProcess/YaoKong ==
  note: 上坡辅助系统(Hill-start Assist Control，HAC)
  mode_dem : Inport
  acc_dem : Inport  Port=2
  steer_dem : Inport  Port=3
  brake_dem : Inport  Port=4
  brake_emerg : Inport  Port=5
  HAC : Inport  Port=6
  Bus Creator : BusCreator  Inputs=6
  YaoKong_dem : Outport
  wires:
  steer_dem/1 -> Bus Creator/3  "steer_dem"
  acc_dem/1 -> Bus Creator/2  "acc_dem"
  brake_dem/1 -> Bus Creator/4  "brake_dem"
  mode_dem/1 -> Bus Creator/1  "mode_dem"
  Bus Creator/1 -> YaoKong_dem/1  "YaoKong"
  brake_emerg/1 -> Bus Creator/5  "brake_emerg"
  HAC/1 -> Bus Creator/6  "HAC"

== system DDCU_wxt_v02_forA_LabviewV01/MainControl/SendOutPrepare ==
  com_dem : Inport
  Data Store Write : DataStoreWrite  DataStoreName=M1Enable
  Data Store Write1 : DataStoreWrite  DataStoreName=M1Mode
  Data Store Write10 : DataStoreWrite  DataStoreName=M3Drive
  Data Store Write11 : DataStoreWrite  DataStoreName=M3TorqueSet
  Data Store Write12 : DataStoreWrite  DataStoreName=M3SpeedSet
  Data Store Write13 : DataStoreWrite  DialogController=Simulink.DDGSource  DataStoreName=M3TrqLimit
  Data Store Write14 : DataStoreWrite  DataStoreName=M3SpeedLimit
  Data Store Write15 : DataStoreWrite  DataStoreName=MCU2HeartBeat
  Data Store Write16 : DataStoreWrite  DataStoreName=M2Enable
  Data Store Write17 : DataStoreWrite  DataStoreName=M2Mode
  Data Store Write18 : DataStoreWrite  DataStoreName=M2Drive
  Data Store Write19 : DataStoreWrite  DataStoreName=M2TorqueSet
  Data Store Write2 : DataStoreWrite  DataStoreName=M1Drive
  Data Store Write20 : DataStoreWrite  DataStoreName=M2SpeedSet
  Data Store Write21 : DataStoreWrite  DataStoreName=M2TrqLimit
  Data Store Write22 : DataStoreWrite  DataStoreName=M2SpeedLimit
  Data Store Write23 : DataStoreWrite  DataStoreName=M4Drive
  Data Store Write24 : DataStoreWrite  DataStoreName=M4TorqueSet
  Data Store Write25 : DataStoreWrite  DataStoreName=M4SpeedSet
  Data Store Write26 : DataStoreWrite  DataStoreName=M4TrqLimit
  Data Store Write27 : DataStoreWrite  DataStoreName=M4SpeedLimit
  Data Store Write28 : DataStoreWrite  DataStoreName=M4Enable
  Data Store Write29 : DataStoreWrite  DataStoreName=M4Mode
  Data Store Write3 : DataStoreWrite  DataStoreName=M1TorqueSet
  Data Store Write30 : DataStoreWrite  DataStoreName=bra_pre_l
  Data Store Write31 : DataStoreWrite  DataStoreName=bra_pre_r
  Data Store Write4 : DataStoreWrite  DataStoreName=M1SpeedSet
  Data Store Write5 : DataStoreWrite  DataStoreName=M1TrqLimit
  Data Store Write6 : DataStoreWrite  DataStoreName=M1SpeedLimit
  Data Store Write7 : DataStoreWrite  DataStoreName=MCU1HeartBeat
  Data Store Write8 : DataStoreWrite  DataStoreName=M3Enable
  Data Store Write9 : DataStoreWrite  DataStoreName=M3Mode
  Demux : Demux  Outputs=6
  Demux1 : Demux  Outputs=8
  Demux2 : Demux  Outputs=8
  Demux3 : Demux  Outputs=7
  Demux4 : Demux  Outputs=7
  Scope{,1..3} (4 alike) : Scope
      Scope2 settings: SaveName=ScopeData2
      Scope3 settings: SaveName=ScopeData3
  wires:
  Demux/1 -> Demux1/1
  Demux/2 -> Demux2/1
  Demux/3 -> Demux3/1
  Demux/4 -> Demux4/1
  Demux1/3 -> Data Store Write2/1
  Demux1/4 -> Scope/1, Data Store Write3/1
  Demux1/2 -> Data Store Write1/1
  Demux1/5 -> Data Store Write4/1
  Demux1/6 -> Data Store Write5/1
  Demux1/1 -> Data Store Write/1
  Demux1/7 -> Data Store Write6/1
  Demux1/8 -> Data Store Write7/1
  Demux2/7 -> Data Store Write14/1
  Demux2/6 -> Data Store Write13/1
  Demux2/1 -> Data Store Write8/1
  Demux2/8 -> Data Store Write15/1
  Demux2/5 -> Data Store Write12/1
  Demux2/2 -> Data Store Write9/1
  Demux2/4 -> Scope1/1, Data Store Write11/1
  Demux2/3 -> Data Store Write10/1
  Demux3/1 -> Data Store Write16/1
  Demux3/6 -> Data Store Write21/1
  Demux3/7 -> Data Store Write22/1
  Demux3/5 -> Data Store Write20/1
  Demux3/4 -> Scope2/1, Data Store Write19/1
  Demux3/2 -> Data Store Write17/1
  Demux3/3 -> Data Store Write18/1
  Demux4/1 -> Data Store Write28/1
  Demux4/2 -> Data Store Write29/1
  Demux4/3 -> Data Store Write23/1
  Demux4/4 -> Scope3/1, Data Store Write24/1
  Demux4/5 -> Data Store Write25/1
  Demux4/6 -> Data Store Write26/1
  Demux4/7 -> Data Store Write27/1
  Demux/5 -> Data Store Write30/1
  Demux/6 -> Data Store Write31/1
  com_dem/1 -> Demux/1

== system DDCU_wxt_v02_forA_LabviewV01/MainControl/mode_control ==
  mode_dem_out : Inport
  Signals : Inport  Port=2
  Multiport Switch : MultiPortSwitch  DataPortOrder=Zero-based contiguous  Inputs=6
  Park : Subsystem  TreatAsAtomicUnit=on
  Switch Case : SwitchCase  CaseConditions={0,1,2,3,4,5}  ShowDefaultCase=off
  backward : Subsystem  TreatAsAtomicUnit=on
  center_steer : Subsystem  TreatAsAtomicUnit=on
  emergency_stop : Subsystem  TreatAsAtomicUnit=on
  forward : Subsystem  TreatAsAtomicUnit=on
  neutral : Subsystem  TreatAsAtomicUnit=on
  com_dem : Outport
  wires:
  mode_dem_out/1 -> Multiport Switch/1, Switch Case/1
  Signals/1 -> backward/1(Signals), emergency_stop/1(Signals), center_steer/1(Signals), neutral/1(Signals), forward/1(Signals), Park/1(Signals)
  Switch Case/1 -> Park/Action
  Switch Case/6 -> emergency_stop/Action
  Switch Case/5 -> center_steer/Action
  Switch Case/4 -> backward/Action
  Switch Case/3 -> neutral/Action
  Switch Case/2 -> forward/Action
  Park/1(park_dem) -> Multiport Switch/2
  forward/1(forward_dem) -> Multiport Switch/3
  backward/1(backward_dem) -> Multiport Switch/5
  neutral/1(neutral_dem) -> Multiport Switch/4
  center_steer/1(center_steer_dem) -> Multiport Switch/6
  emergency_stop/1(emergency_stop_dem) -> Multiport Switch/7
  Multiport Switch/1 -> com_dem/1

== system DDCU_wxt_v02_forA_LabviewV01/MainControl/mode_switch ==
  Signals : Inport
  Abs{,1..3} (4 alike) : Abs
  Bus Selector : BusSelector  OutputSignals=YaoKong.mode_dem,YaoKong.brake_emerg,DriveMotor.speed_act_lf,DriveMotor.speed_act_lr,DriveMotor.speed_act_rf,DriveMotor.speed_act_rr,IMU.v_act
  Constant1 : Constant  Value=v_thr_park
  Constant2 : Constant  Value=speed_thr_park
  Memory : Memory  InheritSampleTime=on
  mode_switch : MATLAB Function  TreatAsAtomicUnit=on
  mode_dem_out : Outport
  wires:
  Memory/1 -> mode_switch/10(mode_dem_out_pre)
  Signals/1 -> Bus Selector/1
  Bus Selector/3 -> Abs/1  "<speed_act_lf>"
  Bus Selector/2 -> mode_switch/2(brake_emerg)  "<brake_emerg>"
  Bus Selector/1 -> mode_switch/1(mode_dem)  "<mode_dem>"
  Bus Selector/5 -> Abs2/1  "<speed_act_rf>"
  Bus Selector/4 -> Abs1/1  "<speed_act_lr>"
  Bus Selector/6 -> Abs3/1  "<speed_act_rr>"
  Bus Selector/7 -> mode_switch/7(v_act)  "<v_act>"
  mode_switch/1(mode_dem_out) -> mode_dem_out/1, Memory/1
  Constant2/1 -> mode_switch/9(speed_thr_park)
  Constant1/1 -> mode_switch/8(v_thr_park)
  Abs/1 -> mode_switch/3(speed_act_lf)
  Abs1/1 -> mode_switch/4(speed_act_lr)
  Abs2/1 -> mode_switch/5(speed_act_rf)
  Abs3/1 -> mode_switch/6(speed_act_rr)

== system DDCU_wxt_v02_forA_LabviewV01/OutputSignalProcess/VCU_ESC ==
  VVMS_BrkSts_flg_in : Inport
  VVMS_ParkSts_flg_in : Inport  Port=2
  VVMS_BrkPSetLe_MPa_in : Inport  Port=3
  VVMS_BrkPSetRi_MPa_in : Inport  Port=4
  Conv{1..8} (8 alike) : DataTypeConversion
  VCU_ESC_DLC : Constant  Value=8  OutDataTypeStr=uint8
  VCU_ESC_DLC_Out : Terminator
  VCU_ESC_ID : Constant  Value=2364992240  OutDataTypeStr=single
  VCU_ESC_ID_Out : Terminator
  VCU_ESC_mux : Mux  Inputs=8
  VVMS_BrkPSetLe_MPa : Subsystem
  VVMS_BrkPSetRi_MPa : Subsystem
  VVMS_BrkSts_flg : Subsystem
  VVMS_ParkSts_flg : Subsystem
  or{1..8} (8 alike) : simulink/Logic and Bit Operations/Bitwise Operator  logicop=OR  UseBitMask=off  NumInputPorts=4  BitMask=bin2dec('11011001')  BitMaskRealWorld=Stored Integer
  output : Outport
  wires:
  VCU_ESC_mux/1 -> output/1
  VVMS_BrkSts_flg/1(output1) -> or1/1
  VVMS_BrkSts_flg/2(output2) -> or2/1
  VVMS_BrkSts_flg/3(output3) -> or3/1
  VVMS_BrkSts_flg/4(output4) -> or4/1
  VVMS_BrkSts_flg/5(output5) -> or5/1
  VVMS_BrkSts_flg/6(output6) -> or6/1
  VVMS_BrkSts_flg/7(output7) -> or7/1
  VVMS_BrkSts_flg/8(output8) -> or8/1
  VVMS_ParkSts_flg/1(output1) -> or1/2
  VVMS_ParkSts_flg/2(output2) -> or2/2
  VVMS_ParkSts_flg/3(output3) -> or3/2
  VVMS_ParkSts_flg/4(output4) -> or4/2
  VVMS_ParkSts_flg/5(output5) -> or5/2
  VVMS_ParkSts_flg/6(output6) -> or6/2
  VVMS_ParkSts_flg/7(output7) -> or7/2
  VVMS_ParkSts_flg/8(output8) -> or8/2
  VVMS_BrkPSetRi_MPa/1(output1) -> or1/3
  VVMS_BrkPSetRi_MPa/2(output2) -> or2/3
  VVMS_BrkPSetRi_MPa/3(output3) -> or3/3
  VVMS_BrkPSetRi_MPa/4(output4) -> or4/3
  VVMS_BrkPSetRi_MPa/5(output5) -> or5/3
  VVMS_BrkPSetRi_MPa/6(output6) -> or6/3
  VVMS_BrkPSetRi_MPa/7(output7) -> or7/3
  VVMS_BrkPSetRi_MPa/8(output8) -> or8/3
  VVMS_BrkPSetLe_MPa/1(output1) -> or1/4
  VVMS_BrkPSetLe_MPa/2(output2) -> or2/4
  VVMS_BrkPSetLe_MPa/3(output3) -> or3/4
  VVMS_BrkPSetLe_MPa/4(output4) -> or4/4
  VVMS_BrkPSetLe_MPa/5(output5) -> or5/4
  VVMS_BrkPSetLe_MPa/6(output6) -> or6/4
  VVMS_BrkPSetLe_MPa/7(output7) -> or7/4
  VVMS_BrkPSetLe_MPa/8(output8) -> or8/4
  or1/1 -> Conv1/1
  Conv1/1 -> VCU_ESC_mux/1
  or2/1 -> Conv2/1
  Conv2/1 -> VCU_ESC_mux/2
  or3/1 -> Conv3/1
  Conv3/1 -> VCU_ESC_mux/3
  or4/1 -> Conv4/1
  Conv4/1 -> VCU_ESC_mux/4
  or5/1 -> Conv5/1
  Conv5/1 -> VCU_ESC_mux/5
  or6/1 -> Conv6/1
  Conv6/1 -> VCU_ESC_mux/6
  or7/1 -> Conv7/1
  Conv7/1 -> VCU_ESC_mux/7
  or8/1 -> Conv8/1
  Conv8/1 -> VCU_ESC_mux/8
  VCU_ESC_ID/1 -> VCU_ESC_ID_Out/1
  VCU_ESC_DLC/1 -> VCU_ESC_DLC_Out/1
  VVMS_BrkSts_flg_in/1 -> VVMS_BrkSts_flg/1(VVMS_BrkSts_flg)
  VVMS_ParkSts_flg_in/1 -> VVMS_ParkSts_flg/1(VVMS_ParkSts_flg)
  VVMS_BrkPSetRi_MPa_in/1 -> VVMS_BrkPSetRi_MPa/1(VVMS_BrkPSetRi_MPa)
  VVMS_BrkPSetLe_MPa_in/1 -> VVMS_BrkPSetLe_MPa/1(VVMS_BrkPSetLe_MPa)

== system DDCU_wxt_v02_forA_LabviewV01/OutputSignalProcess/VCU_MCU1 ==
  M1Enable_in : Inport
  M1Mode_in : Inport  Port=2
  M1Drive_in : Inport  Port=3
  M1TorqueSet_in : Inport  Port=4
  M1SpeedLimit_in : Inport  Port=5
  M2Enable_in : Inport  Port=6
  M2Mode_in : Inport  Port=7
  M2Drive_in : Inport  Port=8
  M2TorqueSet_in : Inport  Port=9
  M2SpeedLimit_in : Inport  Port=10
  MCU1HeartBeat_in : Inport  Port=11
  Conv{1..8} (8 alike) : DataTypeConversion
  M1Drive : Subsystem
  M1Enable : Subsystem
  M1Mode : Subsystem
  M1SpeedLimit : Subsystem
  M1TorqueSet : Subsystem
  M2Drive : Subsystem
  M2Enable : Subsystem
  M2Mode : Subsystem
  M2SpeedLimit : Subsystem
  M2TorqueSet : Subsystem
  MCU1HeartBeat : Subsystem
  VCU_MCU1_DLC : Constant  Value=8  OutDataTypeStr=uint8
  VCU_MCU1_DLC_Out : Terminator
  VCU_MCU1_ID : Constant  Value=2348937217  OutDataTypeStr=single
  VCU_MCU1_ID_Out : Terminator
  VCU_MCU1_mux : Mux  Inputs=8
  or{1..8} (8 alike) : simulink/Logic and Bit Operations/Bitwise Operator  logicop=OR  UseBitMask=off  NumInputPorts=11  BitMask=bin2dec('11011001')  BitMaskRealWorld=Stored Integer
  output : Outport
  wires:
  VCU_MCU1_mux/1 -> output/1
  MCU1HeartBeat/1(output1) -> or1/1
  MCU1HeartBeat/2(output2) -> or2/1
  MCU1HeartBeat/3(output3) -> or3/1
  MCU1HeartBeat/4(output4) -> or4/1
  MCU1HeartBeat/5(output5) -> or5/1
  MCU1HeartBeat/6(output6) -> or6/1
  MCU1HeartBeat/7(output7) -> or7/1
  MCU1HeartBeat/8(output8) -> or8/1
  M2TorqueSet/1(output1) -> or1/2
  M2TorqueSet/2(output2) -> or2/2
  M2TorqueSet/3(output3) -> or3/2
  M2TorqueSet/4(output4) -> or4/2
  M2TorqueSet/5(output5) -> or5/2
  M2TorqueSet/6(output6) -> or6/2
  M2TorqueSet/7(output7) -> or7/2
  M2TorqueSet/8(output8) -> or8/2
  M2SpeedLimit/1(output1) -> or1/3
  M2SpeedLimit/2(output2) -> or2/3
  M2SpeedLimit/3(output3) -> or3/3
  M2SpeedLimit/4(output4) -> or4/3
  M2SpeedLimit/5(output5) -> or5/3
  M2SpeedLimit/6(output6) -> or6/3
  M2SpeedLimit/7(output7) -> or7/3
  M2SpeedLimit/8(output8) -> or8/3
  M2Mode/1(output1) -> or1/4
  M2Mode/2(output2) -> or2/4
  M2Mode/3(output3) -> or3/4
  M2Mode/4(output4) -> or4/4
  M2Mode/5(output5) -> or5/4
  M2Mode/6(output6) -> or6/4
  M2Mode/7(output7) -> or7/4
  M2Mode/8(output8) -> or8/4
  M2Enable/1(output1) -> or1/5
  M2Enable/2(output2) -> or2/5
  M2Enable/3(output3) -> or3/5
  M2Enable/4(output4) -> or4/5
  M2Enable/5(output5) -> or5/5
  M2Enable/6(output6) -> or6/5
  M2Enable/7(output7) -> or7/5
  M2Enable/8(output8) -> or8/5
  M2Drive/1(output1) -> or1/6
  M2Drive/2(output2) -> or2/6
  M2Drive/3(output3) -> or3/6
  M2Drive/4(output4) -> or4/6
  M2Drive/5(output5) -> or5/6
  M2Drive/6(output6) -> or6/6
  M2Drive/7(output7) -> or7/6
  M2Drive/8(output8) -> or8/6
  M1TorqueSet/1(output1) -> or1/7
  M1TorqueSet/2(output2) -> or2/7
  M1TorqueSet/3(output3) -> or3/7
  M1TorqueSet/4(output4) -> or4/7
  M1TorqueSet/5(output5) -> or5/7
  M1TorqueSet/6(output6) -> or6/7
  M1TorqueSet/7(output7) -> or7/7
  M1TorqueSet/8(output8) -> or8/7
  M1SpeedLimit/1(output1) -> or1/8
  M1SpeedLimit/2(output2) -> or2/8
  M1SpeedLimit/3(output3) -> or3/8
  M1SpeedLimit/4(output4) -> or4/8
  M1SpeedLimit/5(output5) -> or5/8
  M1SpeedLimit/6(output6) -> or6/8
  M1SpeedLimit/7(output7) -> or7/8
  M1SpeedLimit/8(output8) -> or8/8
  M1Mode/1(output1) -> or1/9
  M1Mode/2(output2) -> or2/9
  M1Mode/3(output3) -> or3/9
  M1Mode/4(output4) -> or4/9
  M1Mode/5(output5) -> or5/9
  M1Mode/6(output6) -> or6/9
  M1Mode/7(output7) -> or7/9
  M1Mode/8(output8) -> or8/9
  M1Enable/1(output1) -> or1/10
  M1Enable/2(output2) -> or2/10
  M1Enable/3(output3) -> or3/10
  M1Enable/4(output4) -> or4/10
  M1Enable/5(output5) -> or5/10
  M1Enable/6(output6) -> or6/10
  M1Enable/7(output7) -> or7/10
  M1Enable/8(output8) -> or8/10
  M1Drive/1(output1) -> or1/11
  M1Drive/2(output2) -> or2/11
  M1Drive/3(output3) -> or3/11
  M1Drive/4(output4) -> or4/11
  M1Drive/5(output5) -> or5/11
  M1Drive/6(output6) -> or6/11
  M1Drive/7(output7) -> or7/11
  M1Drive/8(output8) -> or8/11
  or1/1 -> Conv1/1
  Conv1/1 -> VCU_MCU1_mux/1
  or2/1 -> Conv2/1
  Conv2/1 -> VCU_MCU1_mux/2
  or3/1 -> Conv3/1
  Conv3/1 -> VCU_MCU1_mux/3
  or4/1 -> Conv4/1
  Conv4/1 -> VCU_MCU1_mux/4
  or5/1 -> Conv5/1
  Conv5/1 -> VCU_MCU1_mux/5
  or6/1 -> Conv6/1
  Conv6/1 -> VCU_MCU1_mux/6
  or7/1 -> Conv7/1
  Conv7/1 -> VCU_MCU1_mux/7
  or8/1 -> Conv8/1
  Conv8/1 -> VCU_MCU1_mux/8
  VCU_MCU1_ID/1 -> VCU_MCU1_ID_Out/1
  VCU_MCU1_DLC/1 -> VCU_MCU1_DLC_Out/1
  MCU1HeartBeat_in/1 -> MCU1HeartBeat/1(MCU1HeartBeat)
  M2TorqueSet_in/1 -> M2TorqueSet/1(M2TorqueSet)
  M2SpeedLimit_in/1 -> M2SpeedLimit/1(M2SpeedLimit)
  M2Mode_in/1 -> M2Mode/1(M2Mode)
  M2Enable_in/1 -> M2Enable/1(M2Enable)
  M2Drive_in/1 -> M2Drive/1(M2Drive)
  M1TorqueSet_in/1 -> M1TorqueSet/1(M1TorqueSet)
  M1SpeedLimit_in/1 -> M1SpeedLimit/1(M1SpeedLimit)
  M1Mode_in/1 -> M1Mode/1(M1Mode)
  M1Enable_in/1 -> M1Enable/1(M1Enable)
  M1Drive_in/1 -> M1Drive/1(M1Drive)
